simulink model "ThisAzzIsOnFire"  (R2015a)
settings: Solver=ode45  StartTime=0.0  StopTime=0.5  RelTol=1e-3
libraries: simulink x1
settings Model: Creator=Alunos  LastModifiedBy=miguel

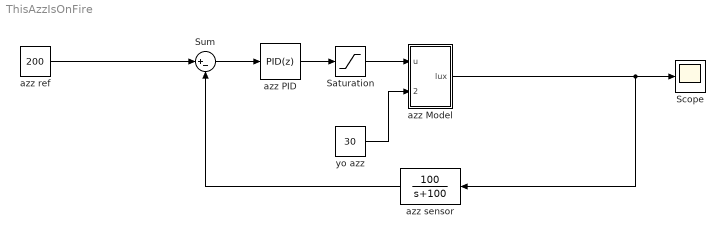
== system ThisAzzIsOnFire ==
  Saturation : Saturate  UpperLimit=5  LowerLimit=0
  Scope : Scope
  Sum : Sum  Inputs=|+-
  azz Model : Subsystem
  azz PID : simulink/Continuous/PID Controller  Controller=PID  TimeDomain=Discrete-time  SampleTime=0.2  IntegratorMethod=Forward Euler  FilterMethod=Forward Euler  Form=Parallel  UseFilter=off  ControllerParametersSource=internal  P=0.00119037240993272  I=0.00595186204966358  D=5.95186204966358e-05  N=320.85434950626  InitialConditionSource=internal  InitialConditionForIntegrator=0  InitialConditionForFilter=0  ExternalReset=none  LimitOutput=off  UpperSaturationLimit=inf  LowerSaturationLimit=-inf  LinearizeAsGain=on  AntiWindupMode=none  Kb=1  TrackingMode=off  Kt=1  PParamMin=[]  PParamMax=[]  IParamMin=[]  IParamMax=[]  DParamMin=[]  DParamMax=[]  NParamMin=[]  NParamMax=[]  KbParamMin=[]  KbParamMax=[]  KtParamMin=[]  KtParamMax=[]  POutMin=[]  POutMax=[]  IOutMin=[]  IOutMax=[]  DOutMin=[]  DOutMax=[]  NOutMin=[]  NOutMax=[]  KbOutMin=[]  KbOutMax=[]  KtOutMin=[]  KtOutMax=[]  IntegratorOutMin=[]  IntegratorOutMax=[]  FilterOutMin=[]  FilterOutMax=[]  SumOutMin=[]  SumOutMax=[]  SumI1OutMin=[]  SumI1OutMax=[]  SumI2OutMin=[]  SumI2OutMax=[]  SumI3OutMin=[]  SumI3OutMax=[]  SumDOutMin=[]  SumDOutMax=[]  SaturationOutMin=[]  SaturationOutMax=[]  IntegratorContinuousStateAttributes=''  IntegratorStateMustResolveToSignalObject=off  IntegratorRTWStateStorageClass=Auto  FilterContinuousStateAttributes=''  FilterStateMustResolveToSignalObject=off  FilterRTWStateStorageClass=Auto  DifferentiatorICPrevScaledInput=0  DifferentiatorOutMin=[]  DifferentiatorOutMax=[]
  azz ref : Constant  Value=200
  azz sensor : TransferFcn  Numerator=[100]  Denominator=[1 100]
  yo azz : Constant  Value=30
  wires:
  azz sensor/1 -> Sum/2
  Sum/1 -> azz PID/1
  azz ref/1 -> Sum/1
  yo azz/1 -> azz Model/2(teta)
  azz Model/1(lux) -> azz sensor/1, Scope/1
  Saturation/1 -> azz Model/1(u)
  azz PID/1 -> Saturation/1

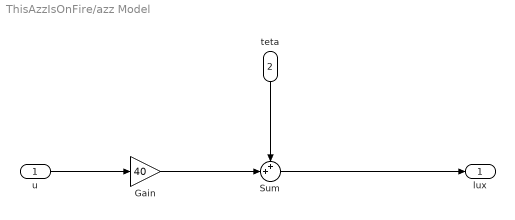
== system ThisAzzIsOnFire/azz Model ==
  u : Inport
  teta : Inport  Port=2
  Gain : Gain  Gain=40
  Sum : Sum  Inputs=++|
  lux : Outport
  wires:
  teta/1 -> Sum/1
  Sum/1 -> lux/1
  Gain/1 -> Sum/2
  u/1 -> Gain/1
